simulink model "Simulink_Discreate_Test_Model"  (R2018a)
settings: Solver=ode15s  StartTime=0.0  StopTime=7  FixedStep=0.0001  RelTol=1e-3  EnableMultiTasking=on
libraries: discretizing x6
settings Model: Creator=user  LastModifiedBy=user
settings SolverCC: ConcurrentTasks=on  AutoInsertRateTranBlk=on
settings DataIOCC: SaveFormat=StructureWithTime  SaveState=on  SignalLoggingName=logsOut
settings OptimizationCC: BlockReduction=off  BooleanDataType=off  OptimizeBlockIOStorage=off  BufferReuse=off  GlobalBufferReuse=off  ExpressionFolding=off  LocalBlockOutputs=off  InitFltsAndDblsToZero=on  OptimizeDataStoreBuffers=off  BusAssignmentInplaceUpdate=off
settings DebuggingCC: SaveWithParameterizedLinksMsg=none  UnderspecifiedInitializationDetection=Classic  MergeDetectMultiDrivingBlocksExec=none  CheckExecutionContextPreStartOutputMsg=on  CheckExecutionContextRuntimeOutputMsg=on  SignalResolutionControl=TryResolveAllWithWarning  SFUnexpectedBacktrackingDiag=warning  SFNoUnconditionalDefaultTransitionDiag=warning  SFExecutionAtInitializationDiag=none
settings HardwareCC: ProdBitPerPointer=32  ProdBitPerSizeT=32  ProdBitPerPtrDiffT=32  ProdLargestAtomicFloat=None  ProdWordSize=32  ProdLongLongMode=on  ProdHWDeviceType=Generic->32-bit x86 compatible
settings ModelReferenceCC: PropagateSignalLabelsOutOfModel=off
settings RTWCC: SystemTargetFile=slrt.tlc  TemplateMakefile=slrt_default_tmf  Description=Simulink Real-Time  CodeExecutionProfiling=on  RTWCompilerOptimization=on
settings CodeAppCC: StateflowObjectComments=on
settings SimulinkRealTimeCC: SupportVariableSizeSignals=on  RL32LogTETModifier=off  xPCConcurrentTasks=on
settings ConfigComp: CovMetricSettings=dw  CovHtmlReporting=on  CovSaveCumulativeToWorkspaceVar=on  CovSaveSingleToWorkspaceVar=on  CovExternalEMLEnable=off  CovSFcnEnable=off

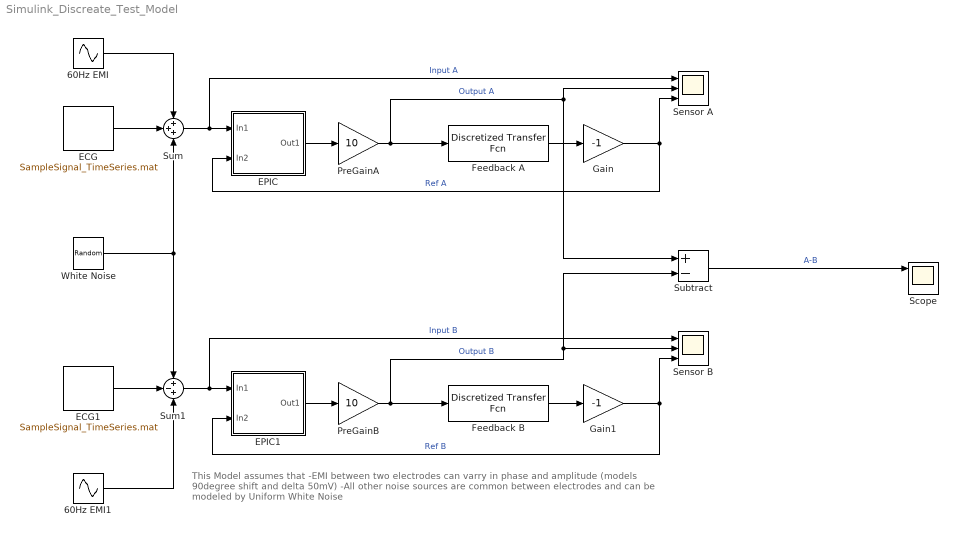
== system Simulink_Discreate_Test_Model ==
  note: This Model assumes that
      | -EMI between two electrodes can varry in phase and amplitude (models 90degree shift and delta 50mV)
      | -All other noise sources are common between electrodes and can be modeled by Uniform White Noise
  60Hz EMI : Sin  Amplitude=0.3  Frequency=377  SampleTime=0.0001
  60Hz EMI1 : Sin  Amplitude=0.35  Frequency=377  Phase=1.97  SampleTime=0.0001
  ECG : FromFile  FileName=SampleSignal_TimeSeries.mat  SampleTime=0
  ECG1 : FromFile  FileName=SampleSignal_TimeSeries.mat  SampleTime=0
  EPIC : Subsystem
  EPIC1 : Subsystem
  Feedback A : discretizing/Discretized Transfer Fcn  Numerator=[1.09 210 25900 59800]  Denominator=[1 19.9 118000 1530]  AbsTol=auto  SampleTime=0.00001  method=matched  Wc=1
  Feedback B : discretizing/Discretized Transfer Fcn  Numerator=[1.09 210 25900 59800]  Denominator=[1 19.9 118000 1530]  AbsTol=auto  SampleTime=0.00001  method=matched  Wc=1
  Gain : Gain  Gain=-1  SaturateOnIntegerOverflow=on  OutDataTypeStr=Inherit: Same as input  ParamDataTypeStr=Inherit: Same as input
  Gain1 : Gain  Gain=-1  SaturateOnIntegerOverflow=on  OutDataTypeStr=Inherit: Same as input  ParamDataTypeStr=Inherit: Same as input
  PreGainA : Gain  Gain=10  OutMin=-5  OutMax=5  SaturateOnIntegerOverflow=on  OutDataTypeStr=Inherit: Same as input  ParamDataTypeStr=Inherit: Same as input
  PreGainB : Gain  Gain=10  OutMin=-5  OutMax=5  SaturateOnIntegerOverflow=on  OutDataTypeStr=Inherit: Same as input  ParamDataTypeStr=Inherit: Same as input
  Scope : Scope  NumInputPorts=3
  Sensor A : Scope  NumInputPorts=3
  Sensor B : Scope  NumInputPorts=3
  Subtract : Sum  Inputs=+-
  Sum : Sum  Inputs=+++
  Sum1 : Sum  Inputs=+-+
  White Noise : UniformRandomNumber  Minimum=-0.1  Maximum=0.1  SampleTime=0.0001
  wires:
  Gain/1 -> Sensor A/3, EPIC/2(In2)  "Ref A"
  EPIC/1(Out1) -> PreGainA/1
  Feedback A/1 -> Gain/1
  ECG/1 -> Sum/2
  PreGainA/1 -> Feedback A/1, Subtract/1, Sensor A/2  "Output A"
  Sum/1 -> Sensor A/1, EPIC/1(In1)  "Input A"
  Sum1/1 -> Sensor B/1, EPIC1/1(In1)  "Input B"
  PreGainB/1 -> Feedback B/1, Sensor B/2, Subtract/2  "Output B"
  EPIC1/1(Out1) -> PreGainB/1
  Feedback B/1 -> Gain1/1
  Gain1/1 -> Sensor B/3, EPIC1/2(In2)  "Ref B"
  60Hz EMI/1 -> Sum/1
  60Hz EMI1/1 -> Sum1/3
  ECG1/1 -> Sum1/2
  White Noise/1 -> Sum/3, Sum1/1
  Subtract/1 -> Scope/1  "A-B"

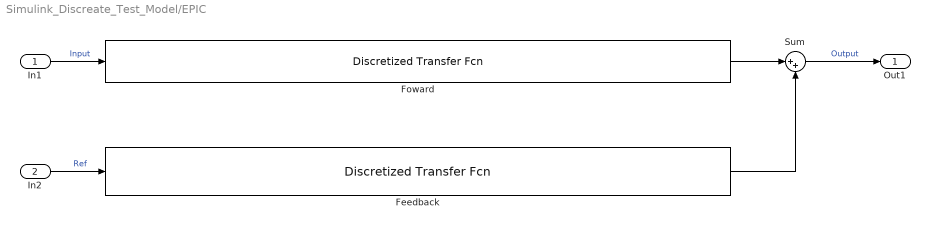
== system Simulink_Discreate_Test_Model/EPIC ==
  In1 : Inport
  In2 : Inport  Port=2
  Feedback : discretizing/Discretized Transfer Fcn  Numerator=[12605.4554063995,23229713663.4924,17234152953470.8,4398216306223.24,3018119162321.11]  Denominator=[1,1423447.52999193,9421519136.03560,6422247005442.77,51913333436888.3,69117764201530.7]  AbsTol=auto  SampleTime=0.00001  method=matched  Wc=1
  Foward : discretizing/Discretized Transfer Fcn  Numerator=[-40596496340164.1,-10055203430225.6,7778571084474.48]  Denominator=[1,3502079.68268747,5589807862084.53,40022776635817.3,58077323621970.0]  AbsTol=auto  SampleTime=0.00001  method=matched  Wc=1
  Sum : Sum  Inputs=|++  OutMin=[-100]  OutMax=[100]
  Out1 : Outport
  wires:
  In1/1 -> Foward/1  "Input"
  Sum/1 -> Out1/1  "Output"
  In2/1 -> Feedback/1  "Ref"
  Foward/1 -> Sum/1
  Feedback/1 -> Sum/2

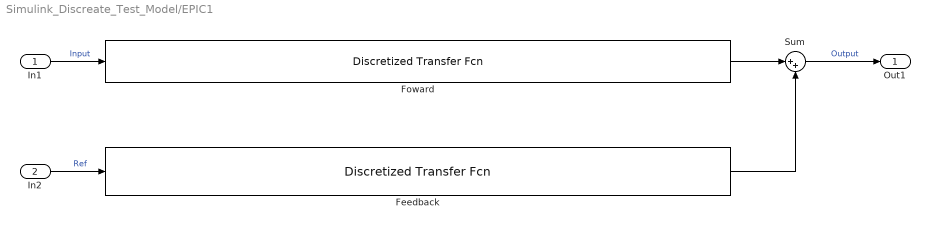
== system Simulink_Discreate_Test_Model/EPIC1 ==
  In1 : Inport
  In2 : Inport  Port=2
  Feedback : discretizing/Discretized Transfer Fcn  Numerator=[12605.4554063995,23229713663.4924,17234152953470.8,4398216306223.24,3018119162321.11]  Denominator=[1,1423447.52999193,9421519136.03560,6422247005442.77,51913333436888.3,69117764201530.7]  AbsTol=auto  SampleTime=0.00001  method=matched  Wc=1
  Foward : discretizing/Discretized Transfer Fcn  Numerator=[0,0,-40596496340164.1,-10055203430225.6,7778571084474.48]  Denominator=[1,3502079.68268747,5589807862084.53,40022776635817.3,58077323621970.0]  AbsTol=auto  SampleTime=0.00001  method=matched  Wc=1
  Sum : Sum  Inputs=|++  OutMin=[-100]  OutMax=[100]
  Out1 : Outport
  wires:
  In1/1 -> Foward/1  "Input"
  Sum/1 -> Out1/1  "Output"
  In2/1 -> Feedback/1  "Ref"
  Foward/1 -> Sum/1
  Feedback/1 -> Sum/2
